simulink model "output_Hinfinty"  (R2023a)
settings: Solver=VariableStepAuto  StartTime=0.0  StopTime=50  RelTol=1e-3
settings Model: Creator=belov  LastModifiedBy=belov

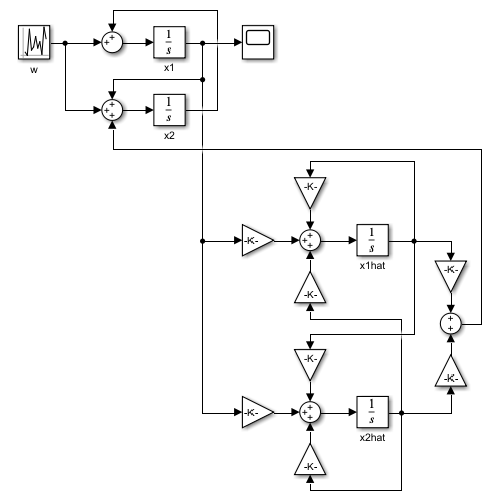
[thumbnail: Simulink's stored preview of the top-level diagram]
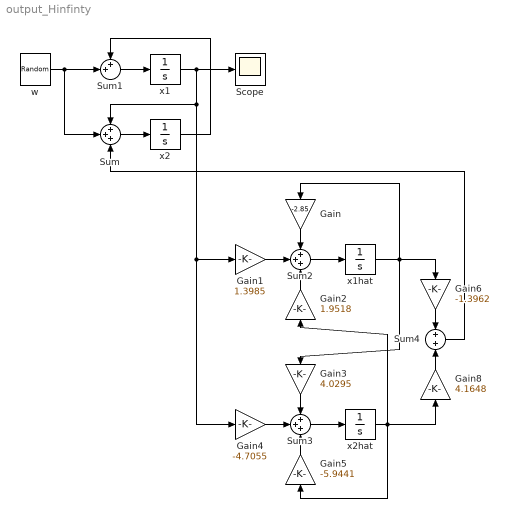
== system output_Hinfinty ==
  Gain : Gain  Gain=-2.85
  Gain1 : Gain  Gain=1.3985
  Gain2 : Gain  Gain=1.9518
  Gain3 : Gain  Gain=4.0295
  Gain4 : Gain  Gain=-4.7055
  Gain5 : Gain  Gain=-5.9441
  Gain6 : Gain  Gain=-1.3962
  Gain8 : Gain  Gain=4.1648
  Scope : Scope
  Sum : Sum  Inputs=+++
  Sum1 : Sum  Inputs=++|
  Sum2 : Sum  Inputs=+++
  Sum3 : Sum  Inputs=+++
  Sum4 : Sum
  w : UniformRandomNumber  Minimum=-0.05  Maximum=0.05  SampleTime=0.1
  x1 : Integrator  InitialCondition=1
  x1hat : Integrator  InitialCondition=1
  x2 : Integrator  InitialCondition=-1
  x2hat : Integrator  InitialCondition=-1
  wires:
  Sum/1 -> x2/1
  Sum1/1 -> x1/1
  x2/1 -> Sum1/1
  w/1 -> Sum/2, Sum1/2
  x1/1 -> Scope/1, Gain4/1, Gain1/1, Sum/1
  Sum2/1 -> x1hat/1
  Gain/1 -> Sum2/1
  Gain1/1 -> Sum2/2
  Gain2/1 -> Sum2/3
  Gain5/1 -> Sum3/3
  Gain4/1 -> Sum3/2
  Gain3/1 -> Sum3/1
  Sum3/1 -> x2hat/1
  x1hat/1 -> Gain6/1, Gain3/1, Gain/1
  x2hat/1 -> Gain5/1, Gain8/1, Gain2/1
  Gain8/1 -> Sum4/2
  Gain6/1 -> Sum4/1
  Sum4/1 -> Sum/3
